simulink model "rRegenDerate"  (R2024b)
settings: configuration reference "STM32H7_Config" (kept outside this file)
settings Model: DataDictionary=Master_Dictionary.sldd  EnableAccessToBaseWorkspace=off  Creator=torni  LastModifiedBy=William
settings ConfigSetRef: SourceName=STM32H7_Config

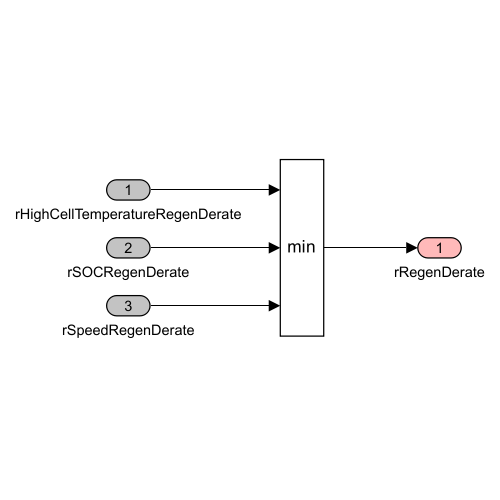
[thumbnail: Simulink's stored preview of the top-level diagram]
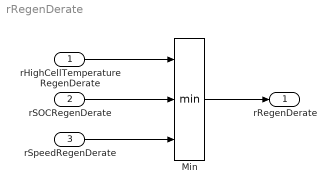
== system rRegenDerate ==
  rHighCellTemperatureRegenDerate : Inport  OutDataTypeStr=double
  rSOCRegenDerate : Inport  Port=2  OutDataTypeStr=double
  rSpeedRegenDerate : Inport  Port=3  OutDataTypeStr=double
  Min : MinMax  Inputs=3
  rRegenDerate : Outport  OutDataTypeStr=double  VectorParamsAs1DForOutWhenUnconnected=off
  wires:
  rHighCellTemperatureRegenDerate/1 -> Min/1
  rSpeedRegenDerate/1 -> Min/3
  Min/1 -> rRegenDerate/1
  rSOCRegenDerate/1 -> Min/2
